simulink model "NCO"  (R2023a)
settings: Solver=VariableStepAuto  StartTime=0.0  StopTime=1  RelTol=1e-3
values from neighbouring files (symbols this model uses):
  hbi = fir2(79,f,mhi)    [fir.m]
libraries: dsphdlfiltering2 x1, dsphdlsigops2 x1
settings Model: Creator=31651  LastModifiedBy=31651
settings OptimizationCC: BlockReduction=off  ConditionallyExecuteInputs=off  DefaultParameterBehavior=Inlined
settings DebuggingCC: AlgebraicLoopMsg=error
settings HardwareCC: ProdBitPerPointer=32  ProdBitPerSizeT=32  ProdBitPerPtrDiffT=32  ProdLargestAtomicFloat=None  ProdIntDivRoundTo=Undefined  ProdEndianess=Unspecified  ProdWordSize=32  ProdHWDeviceType=ASIC/FPGA->ASIC/FPGA  TargetBitPerPointer=64  TargetBitPerSizeT=64  TargetBitPerPtrDiffT=64  TargetLongLongMode=on  TargetIntDivRoundTo=Zero  TargetEndianess=LittleEndian  TargetWordSize=64  TargetHWDeviceType=Custom Processor->MATLAB Host Computer  ProdEqTarget=off

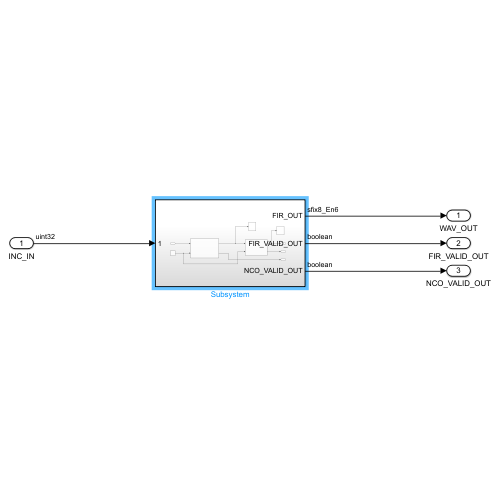
[thumbnail: Simulink's stored preview of the top-level diagram]
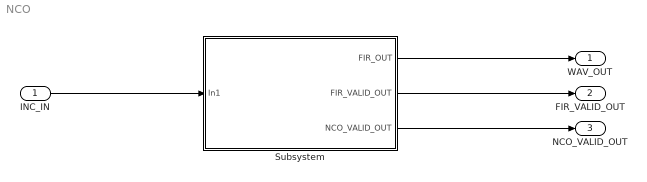
== system NCO ==
  INC_IN : Inport  OutDataTypeStr=uint32
  Subsystem : Subsystem
  WAV_OUT : Outport  VectorParamsAs1DForOutWhenUnconnected=off
  FIR_VALID_OUT : Outport  Port=2  VectorParamsAs1DForOutWhenUnconnected=off
  NCO_VALID_OUT : Outport  Port=3  VectorParamsAs1DForOutWhenUnconnected=off
  wires:
  INC_IN/1 -> Subsystem/1(In1)
  Subsystem/1(FIR_OUT) -> WAV_OUT/1
  Subsystem/2(FIR_VALID_OUT) -> FIR_VALID_OUT/1
  Subsystem/3(NCO_VALID_OUT) -> NCO_VALID_OUT/1

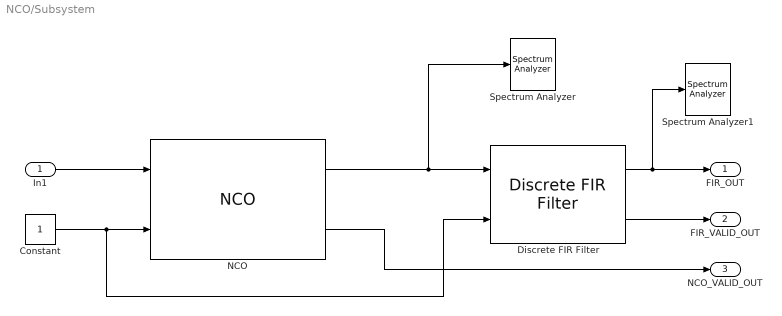
== system NCO/Subsystem ==
  In1 : Inport
  Constant : Constant  OutDataTypeStr=boolean  SampleTime=0.001
  Discrete FIR Filter : dsphdlfiltering2/Discrete FIR Filter  NumeratorSource=Property  Numerator=hbi  NumeratorPrototype=[]  FilterStructure=Direct form systolic  SerializationOption=Minimum number of cycles between valid input samples  NumCycles=2  NumberOfMultipliers=2  SimulateUsing=Code generation  roundingMode=Floor  overflowMode=off  CoefficientsDataTypeStr=Inherit: Same word length as input  OutputDataTypeStr=Inherit: Same word length as input  ResetInputPort=off  HDLGlobalReset=off
  NCO : dsphdlsigops2/NCO  PhaseIncrementSource=Input port  PhaseIncrement=6553  PhaseOffsetSource=Property  PhaseOffset=0  DitherSource=Property  NumDitherBits=4  SamplesPerFrame=1  LUTCompress=off  ResetAction=off  Waveform=Sine  PhasePort=off  SimulateUsing=Code generation  AccumulatorWL=16  PhaseQuantization=on  NumQuantizerAccumulatorBits=12  OutputDataType=Binary point scaling  OutputWL=8  OutputFL=7
      settings: LibrarySourceBlock=dsphdlsrcs2/NCO
  Spectrum Analyzer : SpectrumAnalyzer  WindowPosition=[118.000000,284.000000,800.000000,500.000000,]  Visible=on  ScopeFrameLocation=window  YLimits=[-65.39057723,27.11845593]  ColorLimits=[-20 80]  DefaultConfigurationName=spbscopes.SpectrumAnalyzerBlockCfg  IsFrequencyInputMode=0  FrequencyVectorPort=0  FrequencyVectorFromPort=0  FrequencyInputRBWPort=0  FrequencyInputRBWFromPort=0
  Spectrum Analyzer1 : SpectrumAnalyzer  WindowPosition=[925.000000,257.000000,800.000000,500.000000,]  Visible=on  ScopeFrameLocation=window  YLimits=[-79.87324935,28.52986136]  ColorLimits=[-20 80]  DefaultConfigurationName=spbscopes.SpectrumAnalyzerBlockCfg  IsFrequencyInputMode=0  FrequencyVectorPort=0  FrequencyVectorFromPort=0  FrequencyInputRBWPort=0  FrequencyInputRBWFromPort=0
  FIR_OUT : Outport
  FIR_VALID_OUT : Outport  Port=2
  NCO_VALID_OUT : Outport  Port=3
  wires:
  Discrete FIR Filter/1 -> Spectrum Analyzer1/1, FIR_OUT/1
  Discrete FIR Filter/2 -> FIR_VALID_OUT/1
  Constant/1 -> NCO/2, Discrete FIR Filter/2
  NCO/2 -> NCO_VALID_OUT/1
  NCO/1 -> Spectrum Analyzer/1, Discrete FIR Filter/1
  In1/1 -> NCO/1
